simulink model "simulation_AD_PI_vs_Hinf"  (Simulink 6.3)
settings: Solver=ode15s  StartTime=0.0  StopTime=100  RelTol=1e-6
libraries: cstblocks x4
settings Model: Creator=fromion  LastModifiedBy=xavier.litrico  ExtModeTrigMode=oneshot  ExtModeArmWhenConnect=off  ExtModeAutoUpdateStatusClock=off  BufferReuse=off
settings DataIOCC: InitialState=[]  LimitDataPoints=off  LoadInitialState=on
settings OptimizationCC: BlockReduction=off  BooleanDataType=off  InlineParams=on  BufferReuse=off
settings DebuggingCC: SolverPrmCheckMsg=none
settings HardwareCC: TargetUnknown=on

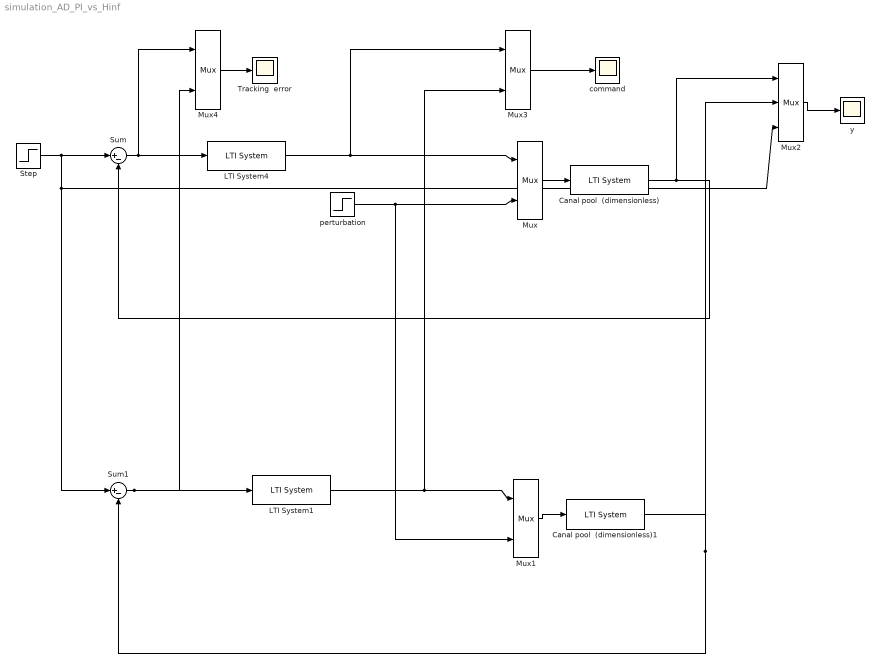
== system simulation_AD_PI_vs_Hinf ==
  Canal pool  (dimensionless) : cstblocks/LTI System  sys=sys_bo_ss  IC=0
  Canal pool  (dimensionless)1 : cstblocks/LTI System  sys=sys_bo_ss  IC=0
  LTI System1 : cstblocks/LTI System  sys=K_PI_ss  IC=0
  LTI System4 : cstblocks/LTI System  sys=K_hinf_ss  IC=0
  Mux{,1,3..4} (4 alike) : Mux  Inputs=2
  Mux2 : Mux  Inputs=3
  Step : Step  SampleTime=0
  Sum : Sum  Inputs=|+-  SaturateOnIntegerOverflow=on  InputSameDT=on
  Sum1 : Sum  Inputs=|+-  SaturateOnIntegerOverflow=on  InputSameDT=on
  Tracking  error : Scope
      settings: SaveName=e  DataFormat=Array
  command : Scope
      settings: SaveName=u  DataFormat=Array
  perturbation : Step  Time=50  SampleTime=0
  y : Scope
      settings: TimeRange=100  SaveName=y  DataFormat=Array  SampleTime=0.1
  wires:
  Sum/1 -> LTI System4/1, Mux4/1
  Canal pool  (dimensionless)/1 -> Sum/2, Mux2/1
  LTI System4/1 -> Mux/1, Mux3/1
  Mux/1 -> Canal pool  (dimensionless)/1
  perturbation/1 -> Mux/2, Mux1/2
  Step/1 -> Sum/1, Sum1/1, Mux2/3
  Sum1/1 -> LTI System1/1, Mux4/2
  Canal pool  (dimensionless)1/1 -> Sum1/2, Mux2/2
  LTI System1/1 -> Mux1/1, Mux3/2
  Mux1/1 -> Canal pool  (dimensionless)1/1
  Mux2/1 -> y/1
  Mux3/1 -> command/1
  Mux4/1 -> Tracking  error/1
